simulink model "wssetq_m"  (Simulink 7.9)
settings: Solver=ode45  SolverMode=SingleTasking  StartTime=0.0  StopTime=999999  MaxStep=10  RelTol=1e-3  AbsTol=1e-3
values from neighbouring files (symbols this model uses):
  U = st_Varia('LongNames')    [wssetq_i.m]
  x0 = []    [wssetq_i.m]    (also in wssetq_s.m = x0)
undefined symbols (not defined in the file or in its folder): B
settings Model: Creator=M.Sparnaaij  LastModifiedBy=M.Sparnaaij
settings DataIOCC: LimitDataPoints=off  SaveOutput=off  SaveTime=off  SignalLoggingName=sigsOut
settings OptimizationCC: BooleanDataType=off
settings DebuggingCC: SaveWithParameterizedLinksMsg=none  SignalResolutionControl=TryResolveAllWithWarning  SolverPrmCheckMsg=none  MultiTaskDSMMsg=warning  MultiTaskCondExecSysMsg=none  StrictBusMsg=None
settings HardwareCC: TargetUnknown=on
settings RTWCC: IncludeERTFirstTime=on
settings GRTTargetCC: CombineOutputUpdateFcns=off  GRTInterface=on

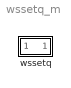
== system wssetq_m ==
  wssetq : Subsystem  Description=wssetq
      mask init:
      | filenaam='.\StimelaData\wssetq_p.mat';
      | 
      | [Pn,Fn,Fext]=Fileprop(filenaam);
      | 
      | errstr = st_UniqName(filenaam,'filenaam=''','SubSystem','OpenFcn');
      | if errstr, error([errstr 'The filename "' filenaam '" is already in use. Choose a different filename.']), end
      | 
      | P = wssetq_p(filenaam);
      | [B,x0,U]=wssetq_i(filenaam);
      settings: OpenFcn=|
      | filenaam='.\StimelaData\wssetq_p.mat';
      | st_ParameterInput('init',gcb,filenaam,'wssetq');
      mask Display:
      | plot(0,0,100,100,[0 20],[50 50],[0 20],[55 55],[80 100],[ 50 50],[80 100],[ 55 55]);
      | patch([20 80 80 20 20],[10 10 90  90 10],[0 0 1])
      | text(50,50,'ws', 'horizontalAlignment', 'center', 'verticalAlignment', 'middle');
      | disp('')

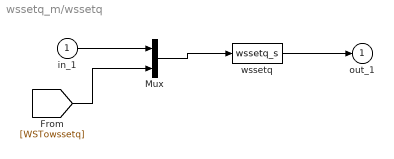
== system wssetq_m/wssetq ==
  in_1 : Inport
  Mux : Mux  Inputs=2
  wssetq : S-Function  FunctionName=wssetq_s  Parameters=B,x0,U,P  EnableBusSupport=off
  out_1 : Outport  InitialOutput=0
  wires:
  wssetq/1 -> out_1/1
  in_1/1 -> Mux/1
  Mux/1 -> wssetq/1
  [WSTowssetq] -> Mux/2
